simulink model "rls_math_model"  (R2021a)
settings: Solver=VariableStepAuto  StartTime=0.0  StopTime=3500  RelTol=1e-3
values from neighbouring files (symbols this model uses):
  A = [-0.0299243213669892 0.0256028069981396 ... (first row only)    [m3007.m]    (also in process_parameters.m = [-1/Tv, 0, 0; real_data_2.m = [-1/Tv, 0, 0; rls_algorithm.m = [-1/Tv, 0, 0)
  A1 = 450    [process_parameters.m]    (also in real_data_2.m; rls_algorithm.m)
  B = [0.00171378115848002; 0]    [m3007.m]    (also in process_parameters.m = [Kv/Tv; 0; 0]; real_data_2.m = [Kv/Tv; 0; 0]; rls_algorithm.m = [Kv/Tv; 0; 0])
  C = [0, 1]    [m3007.m]    (also in process_parameters.m = [0, 0, 1]; real_data_2.m = [0, 0, 1]; rls_algorithm.m = [0, 0, 1])
  delta_xv = 25    [process_parameters.m]    (also in real_data_2.m; rls_algorithm.m)
  g = 981    [process_parameters.m]    (also in real_data_2.m; rls_algorithm.m)
  h10 = data.WaterLevelTank1(start_index)    [m3007.m]    (also in process_parameters.m = 4.69; real_data_2.m = 4.69; rls_algorithm.m = 4.69)
  h20 = data.WaterLevelTank2(start_index)    [m3007.m]    (also in process_parameters.m = 3.39; real_data_2.m = 3.39; rls_algorithm.m = 3.39)
  K12A = K3*A1/sqrt(2*g)    [process_parameters.m]    (also in real_data_2.m; rls_algorithm.m)
  K12B = K2*A1/sqrt(2*g)    [process_parameters.m]    (also in real_data_2.m; rls_algorithm.m)
  K1d = K4*A1/sqrt(2*g)    [process_parameters.m]    (also in real_data_2.m; rls_algorithm.m)
  K2d = K4*A1/sqrt(2*g)    [process_parameters.m]    (also in real_data_2.m; rls_algorithm.m)
  Ki = K1*A1/sqrt(2*g)    [process_parameters.m]    (also in real_data_2.m; rls_algorithm.m)
  Kv = 3.0519 + 0.3    (= 3.3519)    [process_parameters.m]    (also in real_data_2.m = 3.2519; rls_algorithm.m = 3.2519)
  qu0 = data.InletFlow(start_index)*(1000/60)    [m3007.m]    (also in process_parameters.m = 93; real_data_2.m = 82; rls_algorithm.m = 82)
  Ts = 0.1    [process_parameters.m]    (also in real_data_2.m = 0.01; rls_algorithm.m)
  Tv = 1.74    [process_parameters.m]    (also in real_data_2.m; rls_algorithm.m)
  xv0 = 25    [process_parameters.m]    (also in real_data_2.m; rls_algorithm.m)
libraries: simulink x3
settings Model: Creator=matij  LastModifiedBy=matij

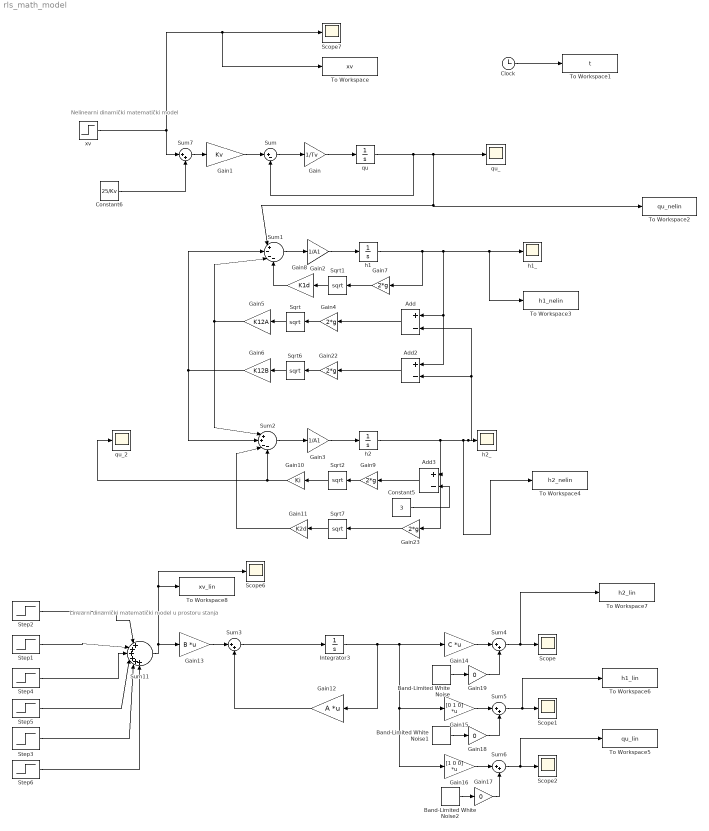
== system rls_math_model ==
  note: Linearni dinamički matematički model u prostoru stanja
  note: Nelinearni dinamički matematički model
  Add : Sum  Inputs=+-
  Add2 : Sum  Inputs=+-
  Add3 : Sum  Inputs=+-
  Band-Limited White Noise : simulink/Sources/Band-Limited White Noise  Cov=[0.0007]  Ts=0.5  seed=[23341]
  Band-Limited White Noise1 : simulink/Sources/Band-Limited White Noise  Cov=[0.0007]  Ts=0.5  seed=[23341]
  Band-Limited White Noise2 : simulink/Sources/Band-Limited White Noise  Cov=[0.00000]  Ts=0.5  seed=[23341]
  Clock : Clock
  Constant5 : Constant  Value=3
  Constant6 : Constant  Value=25/Kv
  Gain : Gain  Gain=1/Tv
  Gain1 : Gain  Gain=Kv
  Gain10 : Gain  Gain=Ki
  Gain11 : Gain  Gain=K2d
  Gain12 : Gain  Gain=A  Multiplication=Matrix(K*u)
  Gain13 : Gain  Gain=B  Multiplication=Matrix(K*u)
  Gain14 : Gain  Gain=C  Multiplication=Matrix(K*u)
  Gain15 : Gain  Gain=[0 1 0]  Multiplication=Matrix(K*u)
  Gain16 : Gain  Gain=[1 0 0]  Multiplication=Matrix(K*u)
  Gain17 : Gain  Gain=0
  Gain18 : Gain  Gain=0
  Gain19 : Gain  Gain=0
  Gain2 : Gain  Gain=1/A1
  Gain{4,7,9,22..23} (5 alike) : Gain  Gain=2*g
  Gain3 : Gain  Gain=1/A1
  Gain5 : Gain  Gain=K12A
  Gain6 : Gain  Gain=K12B
  Gain8 : Gain  Gain=K1d
  Integrator3 : Integrator
  Scope{,1..2,6..7} (5 alike) : Scope
  Sqrt{,1..2,6..7} (5 alike) : Sqrt  SaturateOnIntegerOverflow=on
  Step1 : Step  Time=800  After=-15  SampleTime=0
  Step2 : Step  Time=0.5  After=delta_xv  SampleTime=0
  Step3 : Step  Time=2500  After=+10  SampleTime=0
  Step4 : Step  Time=1410  After=+13  SampleTime=0
  Step5 : Step  Time=1950  After=-18  SampleTime=0
  Step6 : Step  Time=3000  After=-5  SampleTime=0
  Sum : Sum  Inputs=|+-
  Sum1 : Sum  Inputs=|+---
  Sum11 : Sum  Inputs=|++++++
  Sum2 : Sum  Inputs=|++--
  Sum{3..7} (5 alike) : Sum  Inputs=|++
  To Workspace : ToWorkspace  VariableName=xv  SampleTime=Ts
  To Workspace1 : ToWorkspace  VariableName=t  SampleTime=Ts
  To Workspace2 : ToWorkspace  VariableName=qu_nelin  SampleTime=Ts
  To Workspace3 : ToWorkspace  VariableName=h1_nelin  SampleTime=Ts
  To Workspace4 : ToWorkspace  VariableName=h2_nelin  SampleTime=Ts
  To Workspace5 : ToWorkspace  VariableName=qu_lin  SampleTime=Ts
  To Workspace6 : ToWorkspace  VariableName=h1_lin  SampleTime=Ts
  To Workspace7 : ToWorkspace  VariableName=h2_lin  SampleTime=Ts
  To Workspace8 : ToWorkspace  VariableName=xv_lin  SampleTime=Ts
  h1 : Integrator  InitialCondition=h10
  h1_ : Scope
  h2 : Integrator  InitialCondition=h20
  h2_ : Scope
  qu : Integrator  InitialCondition=qu0
  qu_ : Scope
  qu_2 : Scope
  xv : Step  Time=0  Before=xv0  After=xv0+delta_xv  SampleTime=0
  wires:
  Gain/1 -> qu/1
  Gain1/1 -> Sum/1
  Sum/1 -> Gain/1
  h1/1 -> Add2/1, Add/1, To Workspace3/1, h1_/1, Gain7/1
  Sum1/1 -> Gain2/1
  Gain2/1 -> h1/1
  Sum2/1 -> Gain3/1
  Gain3/1 -> h2/1
  Gain4/1 -> Sqrt/1
  Sqrt/1 -> Gain5/1
  Gain6/1 -> Sum1/2, Sum2/2
  Gain5/1 -> Sum1/3, Sum2/1
  Gain7/1 -> Sqrt1/1
  Sqrt1/1 -> Gain8/1
  Gain8/1 -> Sum1/4
  Gain9/1 -> Sqrt2/1
  Sqrt2/1 -> Gain10/1
  Gain10/1 -> qu_2/1, Sum2/4
  Gain11/1 -> Sum2/3
  Sum3/1 -> Integrator3/1
  Gain13/1 -> Sum3/1
  Gain12/1 -> Sum3/2
  Integrator3/1 -> Gain14/1, Gain15/1, Gain16/1, Gain12/1
  Clock/1 -> To Workspace1/1
  qu/1 -> Sum/2, Sum1/1, To Workspace2/1, qu_/1
  h2/1 -> Gain23/1, Add3/1, Add/2, Add2/2, h2_/1, To Workspace4/1
  Constant5/1 -> Add3/2
  Sqrt6/1 -> Gain6/1
  Gain22/1 -> Sqrt6/1
  Sqrt7/1 -> Gain11/1
  Gain23/1 -> Sqrt7/1
  Add/1 -> Gain4/1
  Add2/1 -> Gain22/1
  Add3/1 -> Gain9/1
  xv/1 -> Sum7/1, Scope7/1, To Workspace/1
  Sum7/1 -> Gain1/1
  Constant6/1 -> Sum7/2
  Step2/1 -> Sum11/1
  Sum11/1 -> Scope6/1, To Workspace8/1, Gain13/1
  Step4/1 -> Sum11/3
  Step5/1 -> Sum11/4
  Step3/1 -> Sum11/5
  Step6/1 -> Sum11/6
  Step1/1 -> Sum11/2
  Gain14/1 -> Sum4/1
  Sum4/1 -> Scope/1, To Workspace7/1
  Band-Limited White Noise/1 -> Gain19/1
  Gain15/1 -> Sum5/1
  Sum5/1 -> To Workspace6/1, Scope1/1
  Band-Limited White Noise1/1 -> Gain18/1
  Gain16/1 -> Sum6/1
  Band-Limited White Noise2/1 -> Gain17/1
  Sum6/1 -> To Workspace5/1, Scope2/1
  Gain17/1 -> Sum6/2
  Gain18/1 -> Sum5/2
  Gain19/1 -> Sum4/2
